simulink model "sim12ex5"  (Simulink 4.00)
settings: Solver=ode45  SolverMode=SingleTasking  StartTime=0.0  StopTime=25  MaxStep=.1  RelTol=1e-3  AbsTol=1e-3
settings Model: LastModifiedBy=saadat  SaveTime=off  SaveOutput=off  LimitDataPoints=off  RTWTemplateMakefile=grt_vc.tmf  ExtModeTrigMode=oneshot  ExtModeArmWhenConnect=off

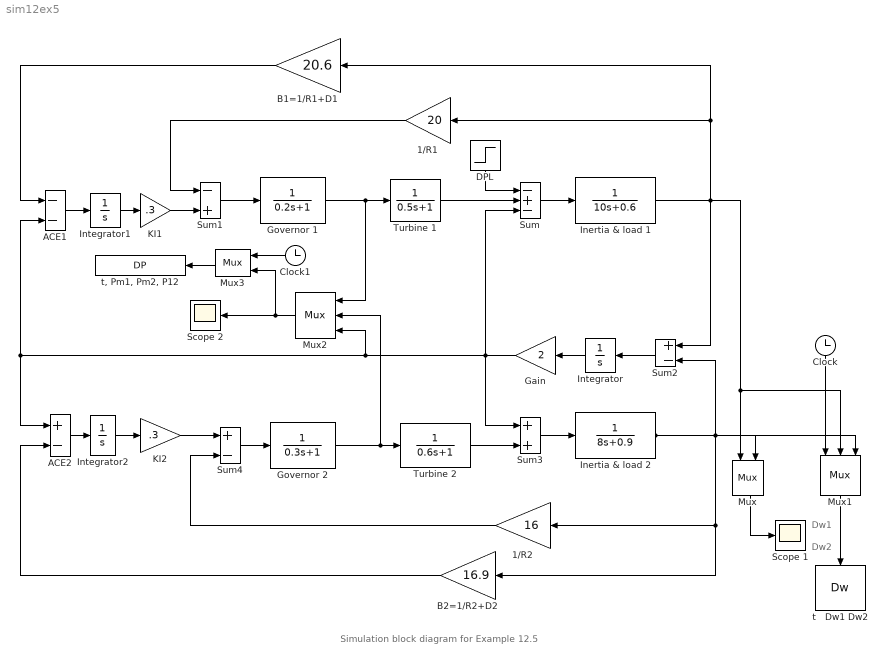
== system sim12ex5 ==
  note: Dw1
  note: Dw2
  note: Simulation block diagram for Example 12.5
  "   Governor 2" : TransferFcn  Numerator=[1]  Denominator="[0.3   1]"  AbsoluteTolerance=auto  Realization=auto
  " Governor 1" : TransferFcn  Numerator=[1]  Denominator="[0.2   1]"  AbsoluteTolerance=auto  Realization=auto
  " Turbine 1" : TransferFcn  Numerator=[1]  Denominator="[0.5  1]"  AbsoluteTolerance=auto  Realization=auto
  1/R1 : Gain  Orientation=left  Gain=20  Multiplication=Element-wise(K.*u)  SaturateOnIntegerOverflow=on
  "1/R2 " : Gain  Orientation=left  Gain=16  Multiplication=Element-wise(K.*u)  SaturateOnIntegerOverflow=on
  ACE1 : Sum  Inputs=--  SaturateOnIntegerOverflow=on
  ACE2 : Sum  Inputs=+-  SaturateOnIntegerOverflow=on
  B1=1/R1+D1 : Gain  Orientation=left  Gain=20.6  Multiplication=Element-wise(K.*u)  SaturateOnIntegerOverflow=on
  B2=1/R2+D2 : Gain  Orientation=left  Gain=16.9  Multiplication=Element-wise(K.*u)  SaturateOnIntegerOverflow=on
  Clock : Clock
      settings: Orientation=down  DisplayTime=off  Decimation=10
  Clock1 : Clock
      settings: DisplayTime=off  Decimation=10
  "DPL " : Step  Orientation=down  Time=0  Before=0  After=0.1875  SampleTime=0
  Gain : Gain  Orientation=left  Gain=2  Multiplication=Element-wise(K.*u)  SaturateOnIntegerOverflow=on
  "Inertia & load 1 " : TransferFcn  Numerator=[1]  Denominator="[10  0.6]"  AbsoluteTolerance=auto  Realization=auto
  Inertia & load 2 : TransferFcn  Numerator=[1]  Denominator="[8  0.9]"  AbsoluteTolerance=auto  Realization=auto
  Integrator : Integrator  Orientation=left  ExternalReset=none  InitialConditionSource=internal  InitialCondition=0  LimitOutput=off  UpperSaturationLimit=inf  LowerSaturationLimit=-inf  ShowSaturationPort=off  ShowStatePort=off  AbsoluteTolerance=auto
  Integrator1 : Integrator  ExternalReset=none  InitialConditionSource=internal  InitialCondition=0  LimitOutput=off  UpperSaturationLimit=inf  LowerSaturationLimit=-inf  ShowSaturationPort=off  ShowStatePort=off  AbsoluteTolerance=auto
  Integrator2 : Integrator  ExternalReset=none  InitialConditionSource=internal  InitialCondition=0  LimitOutput=off  UpperSaturationLimit=inf  LowerSaturationLimit=-inf  ShowSaturationPort=off  ShowStatePort=off  AbsoluteTolerance=auto
  KI1 : Gain  Gain=.3  Multiplication=Element-wise(K.*u)  SaturateOnIntegerOverflow=on
  "KI2 " : Gain  Gain=.3  Multiplication=Element-wise(K.*u)  SaturateOnIntegerOverflow=on
  Mux : Mux  Orientation=down  Inputs=2
      settings: DisplayOption=none
  Mux1 : Mux  Orientation=down  Inputs=3
      settings: DisplayOption=none
  Mux2 : Mux  Orientation=left  Inputs=3
      settings: DisplayOption=none
  Mux3 : Mux  Orientation=left  Inputs=2
      settings: DisplayOption=none
  Scope 1 : Scope
      settings: TickLabels=on  TimeRange=25  YMin=-0.015  YMax=0.005  SaveToWorkspace=off  SaveName=ScopeData  DataFormat=Array  LimitDataPoints=on  MaxDataPoints=5000
  Scope 2 : Scope
      settings: TickLabels=on  TimeRange=25  YMin=-0.1  YMax=0.4  SaveToWorkspace=off  SaveName=ScopeData  DataFormat=Array  LimitDataPoints=on  MaxDataPoints=5000
  Sum : Sum  Inputs=-+-  SaturateOnIntegerOverflow=on
  Sum1 : Sum  Inputs=-+  SaturateOnIntegerOverflow=on
  Sum2 : Sum  Orientation=left  Inputs=+-  SaturateOnIntegerOverflow=on
  Sum3 : Sum  Inputs=++  SaturateOnIntegerOverflow=on
  Sum4 : Sum  Inputs=+-  SaturateOnIntegerOverflow=on
  Turbine 2 : TransferFcn  Numerator=[1]  Denominator="[0.6  1]"  AbsoluteTolerance=auto  Realization=auto
  t   Dw1 Dw2 : ToWorkspace  VariableName=Dw  SampleTime=0  SaveFormat=Array
      settings: Orientation=down  MaxDataPoints=1000
  "t, Pm1, Pm2, P12" : ToWorkspace  VariableName=DP  SampleTime=0  SaveFormat=Array
      settings: MaxDataPoints=1000
  wires:
  " Turbine 1"/1 -> Sum/2
  Sum/1 -> "Inertia & load 1 "/1
  Sum1/1 -> " Governor 1"/1
  "DPL "/1 -> Sum/1
  1/R1/1 -> Sum1/1
  Sum2/1 -> Integrator/1
  Integrator/1 -> Gain/1
  Sum3/1 -> Inertia & load 2/1
  Sum4/1 -> "   Governor 2"/1
  Turbine 2/1 -> Sum3/2
  "1/R2 "/1 -> Sum4/2
  Inertia & load 2/1 -> Mux1/3, Mux/2, "1/R2 "/1, B2=1/R2+D2/1, Sum2/2
  Mux1/1 -> t   Dw1 Dw2/1
  Clock/1 -> Mux1/1
  KI1/1 -> Sum1/2
  Integrator1/1 -> KI1/1
  ACE1/1 -> Integrator1/1
  Integrator2/1 -> "KI2 "/1
  ACE2/1 -> Integrator2/1
  "KI2 "/1 -> Sum4/1
  B1=1/R1+D1/1 -> ACE1/1
  B2=1/R2+D2/1 -> ACE2/2
  Mux/1 -> Scope 1/1
  Gain/1 -> Sum/3, Sum3/1, ACE1/2, ACE2/1, Mux2/3
  " Governor 1"/1 -> " Turbine 1"/1, Mux2/1
  "   Governor 2"/1 -> Turbine 2/1, Mux2/2
  "Inertia & load 1 "/1 -> Sum2/1, 1/R1/1, B1=1/R1+D1/1, Mux/1, Mux1/2
  Mux2/1 -> Scope 2/1, Mux3/2
  Clock1/1 -> Mux3/1
  Mux3/1 -> "t, Pm1, Pm2, P12"/1
